simulink model "CartWithFullSubsystems"  (R2020a)
settings: Solver=VariableStepAuto  StartTime=0.0  StopTime=100  RelTol=1e-3
libraries: robotlib x12
settings Model: EnablePacing=on  Creator=eduar  LastModifiedBy=Ishmael

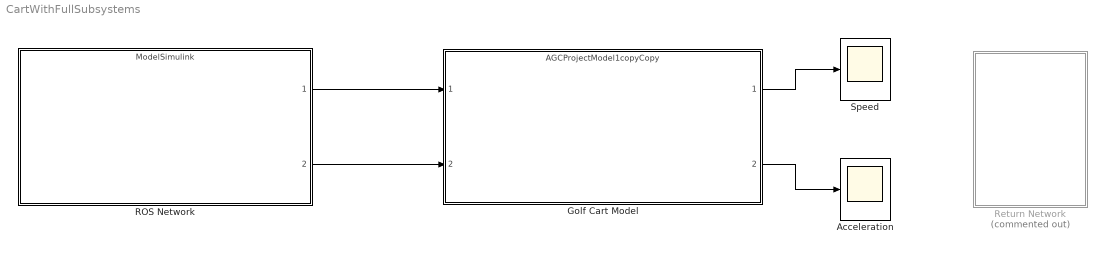
== system CartWithFullSubsystems ==
  Acceleration : Scope
  Golf Cart Model : ModelReference  ModelNameDialog=AGCProjectModel1copyCopy.slx  SimulationMode=Normal  ModelReferenceVersion=1.52
  ROS Network : ModelReference  ModelNameDialog=ModelSimulink.slx  SimulationMode=Normal  ModelReferenceVersion=1.22
  Return Network : Subsystem  Commented=on
  Speed : Scope
  wires:
  Golf Cart Model/1 -> Speed/1
  Golf Cart Model/2 -> Acceleration/1
  ROS Network/1 -> Golf Cart Model/1
  ROS Network/2 -> Golf Cart Model/2

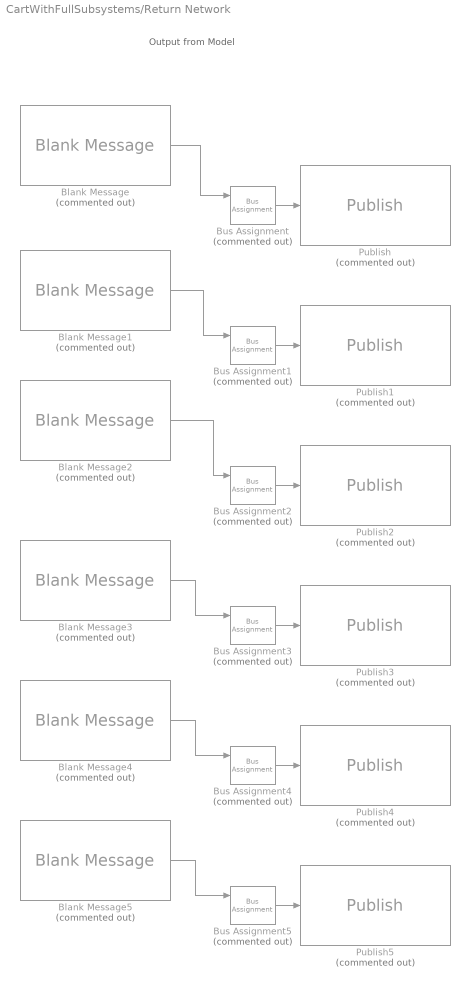
== system CartWithFullSubsystems/Return Network ==
  note: Output from Model
  Blank Message{,1..5} (6 alike) : robotlib/Blank Message  Commented=on  messageClass=Message  entityType=geometry_msgs/Twist  messageType=geometry_msgs/Twist  SampleTime=inf
  Bus Assignment{,1..5} (6 alike) : BusAssignment  Commented=on  AssignedSignals=Linear.X
  Publish : robotlib/Publish  Commented=on  topicSource=Select from ROS network  topic=/Model/PedalPositionReturn  messageType=geometry_msgs/Twist  messageQueueLength=1
  Publish1 : robotlib/Publish  Commented=on  topicSource=Select from ROS network  topic=/Model/SteeringPositionReturn  messageType=geometry_msgs/Twist  messageQueueLength=1
  Publish2 : robotlib/Publish  Commented=on  topicSource=Select from ROS network  topic=/Model/BreakingPositionReturn  messageType=geometry_msgs/Twist  messageQueueLength=1
  Publish3 : robotlib/Publish  Commented=on  topicSource=Select from ROS network  topic=/Model/Acceleration  messageType=geometry_msgs/Twist  messageQueueLength=1
  Publish4 : robotlib/Publish  Commented=on  topicSource=Select from ROS network  topic=/Model/TireAngle  messageType=geometry_msgs/Twist  messageQueueLength=1
  Publish5 : robotlib/Publish  Commented=on  topicSource=Select from ROS network  topic=/Model/Camera  messageType=geometry_msgs/Twist  messageQueueLength=1
  wires:
  Blank Message1/1 -> Bus Assignment1/1
  Blank Message/1 -> Bus Assignment/1
  Bus Assignment1/1 -> Publish1/1
  ? -> Bus Assignment/2
  ? -> Bus Assignment5/2
  Bus Assignment5/1 -> Publish5/1
  Blank Message5/1 -> Bus Assignment5/1
  ? -> Bus Assignment1/2
  ? -> Bus Assignment3/2
  Blank Message4/1 -> Bus Assignment4/1
  Blank Message3/1 -> Bus Assignment3/1
  Bus Assignment/1 -> Publish/1
  ? -> Bus Assignment4/2
  ? -> Bus Assignment2/2
  Bus Assignment4/1 -> Publish4/1
  Blank Message2/1 -> Bus Assignment2/1
  Bus Assignment3/1 -> Publish3/1
  Bus Assignment2/1 -> Publish2/1
